simulink model "gm_uz_pmsm_model_9ph_21b_all_double_vnl"  (R2021b)
settings: Solver=FixedStepAuto  StartTime=0.0  StopTime=0.8  RelTol=1e-3
PreLoadFcn:
  | uz_pmsm_model_9ph_init_parameter
undefined symbols (not defined in the file or in its folder): a, b, c, friction_coefficient, inertia, k_i_d, k_i_q, k_p_d, k_p_q, Kpd, L_d, L_o1, L_o2, L_q, L_x1, L_x2, L_y1, L_y2, L_zero, polepair, psi_pm, R_1, static_friction_torque, Tnd, ts
libraries: hdlsllib x91, simulink x46, hdlmdlgenlib x17, dspsigops x7, slpidlib x2, spsAlphaBetaZerotodq0Lib x1, pid_lib x1, spsdq0toAlphaBetaZeroLib x1
(part 7 of 7)

== system gm_uz_pmsm_model_9ph_21b_all_double_vnl/uz_pmsm_model_9ph/abc_to_dq/abc_to_dq/_adder_MultiplyAdd74 ==
  in0 : Inport  OutDataTypeStr=fixdt(1, 18, 17)  SampleTime=1e-08
  in1 : Inport  Port=2  OutDataTypeStr=fixdt(1, 25, 12)  SampleTime=1e-08
  in2 : Inport  Port=3  OutDataTypeStr=fixdt(1, 25, 12)  SampleTime=1e-08
  globalSchedule : EnablePort  OutDataTypeStr=boolean
  HwModeRegister : Delay  DelayLength=double(1)  InitialCondition=0
  HwModeRegister1 : Delay  DelayLength=double(1)  InitialCondition=0
  HwModeRegister2 : Delay  DelayLength=double(1)  InitialCondition=0
  PipelineRegister : Delay  DelayLength=double(2)  InitialCondition=0
  _adder_MultiplyAdd : hdlsllib/HDL Operations/Multiply-Add  Function=c+(a.*b)  datatype=fixdt(1, 44, 29)  DoSatur=off  FMA=off
      settings: SourceProductBaseCode=SL
  out0 : Outport  OutDataTypeStr=fixdt(1, 44, 29)  SampleTime=1e-08  InitialOutput=0
  wires:
  HwModeRegister2/1 -> _adder_MultiplyAdd/3
  HwModeRegister1/1 -> _adder_MultiplyAdd/2
  HwModeRegister/1 -> _adder_MultiplyAdd/1
  _adder_MultiplyAdd/1 -> PipelineRegister/1
  in2/1 -> HwModeRegister2/1
  in1/1 -> HwModeRegister1/1
  in0/1 -> HwModeRegister/1
  PipelineRegister/1 -> out0/1

== system gm_uz_pmsm_model_9ph_21b_all_double_vnl/uz_pmsm_model_9ph/abc_to_dq/abc_to_dq/_adder_MultiplyAdd75 ==
  in0 : Inport  OutDataTypeStr=fixdt(1, 18, 17)  SampleTime=1e-08
  in1 : Inport  Port=2  OutDataTypeStr=fixdt(1, 25, 12)  SampleTime=1e-08
  in2 : Inport  Port=3  OutDataTypeStr=fixdt(1, 25, 12)  SampleTime=1e-08
  globalSchedule : EnablePort  OutDataTypeStr=boolean
  HwModeRegister : Delay  DelayLength=double(1)  InitialCondition=0
  HwModeRegister1 : Delay  DelayLength=double(1)  InitialCondition=0
  HwModeRegister2 : Delay  DelayLength=double(1)  InitialCondition=0
  PipelineRegister : Delay  DelayLength=double(2)  InitialCondition=0
  _adder_MultiplyAdd : hdlsllib/HDL Operations/Multiply-Add  Function=c+(a.*b)  datatype=fixdt(1, 44, 29)  DoSatur=off  FMA=off
      settings: SourceProductBaseCode=SL
  out0 : Outport  OutDataTypeStr=fixdt(1, 44, 29)  SampleTime=1e-08  InitialOutput=0
  wires:
  HwModeRegister2/1 -> _adder_MultiplyAdd/3
  HwModeRegister1/1 -> _adder_MultiplyAdd/2
  HwModeRegister/1 -> _adder_MultiplyAdd/1
  _adder_MultiplyAdd/1 -> PipelineRegister/1
  in2/1 -> HwModeRegister2/1
  in1/1 -> HwModeRegister1/1
  in0/1 -> HwModeRegister/1
  PipelineRegister/1 -> out0/1

== system gm_uz_pmsm_model_9ph_21b_all_double_vnl/uz_pmsm_model_9ph/abc_to_dq/abc_to_dq/_adder_MultiplyAdd76 ==
  in0 : Inport  OutDataTypeStr=fixdt(1, 18, 17)  SampleTime=1e-08
  in1 : Inport  Port=2  OutDataTypeStr=fixdt(1, 25, 12)  SampleTime=1e-08
  in2 : Inport  Port=3  OutDataTypeStr=fixdt(1, 25, 12)  SampleTime=1e-08
  globalSchedule : EnablePort  OutDataTypeStr=boolean
  HwModeRegister : Delay  DelayLength=double(1)  InitialCondition=0
  HwModeRegister1 : Delay  DelayLength=double(1)  InitialCondition=0
  HwModeRegister2 : Delay  DelayLength=double(1)  InitialCondition=0
  PipelineRegister : Delay  DelayLength=double(2)  InitialCondition=0
  _adder_MultiplyAdd : hdlsllib/HDL Operations/Multiply-Add  Function=c+(a.*b)  datatype=fixdt(1, 44, 29)  DoSatur=off  FMA=off
      settings: SourceProductBaseCode=SL
  out0 : Outport  OutDataTypeStr=fixdt(1, 44, 29)  SampleTime=1e-08  InitialOutput=0
  wires:
  HwModeRegister2/1 -> _adder_MultiplyAdd/3
  HwModeRegister1/1 -> _adder_MultiplyAdd/2
  HwModeRegister/1 -> _adder_MultiplyAdd/1
  _adder_MultiplyAdd/1 -> PipelineRegister/1
  in2/1 -> HwModeRegister2/1
  in1/1 -> HwModeRegister1/1
  in0/1 -> HwModeRegister/1
  PipelineRegister/1 -> out0/1

== system gm_uz_pmsm_model_9ph_21b_all_double_vnl/uz_pmsm_model_9ph/abc_to_dq/abc_to_dq/_adder_MultiplyAdd77 ==
  in0 : Inport  OutDataTypeStr=fixdt(1, 18, 17)  SampleTime=1e-08
  in1 : Inport  Port=2  OutDataTypeStr=fixdt(1, 25, 12)  SampleTime=1e-08
  in2 : Inport  Port=3  OutDataTypeStr=fixdt(1, 25, 12)  SampleTime=1e-08
  globalSchedule : EnablePort  OutDataTypeStr=boolean
  HwModeRegister : Delay  DelayLength=double(1)  InitialCondition=0
  HwModeRegister1 : Delay  DelayLength=double(1)  InitialCondition=0
  HwModeRegister2 : Delay  DelayLength=double(1)  InitialCondition=0
  PipelineRegister : Delay  DelayLength=double(2)  InitialCondition=0
  _adder_MultiplyAdd : hdlsllib/HDL Operations/Multiply-Add  Function=c+(a.*b)  datatype=fixdt(1, 44, 29)  DoSatur=off  FMA=off
      settings: SourceProductBaseCode=SL
  out0 : Outport  OutDataTypeStr=fixdt(1, 44, 29)  SampleTime=1e-08  InitialOutput=0
  wires:
  HwModeRegister2/1 -> _adder_MultiplyAdd/3
  HwModeRegister1/1 -> _adder_MultiplyAdd/2
  HwModeRegister/1 -> _adder_MultiplyAdd/1
  _adder_MultiplyAdd/1 -> PipelineRegister/1
  in2/1 -> HwModeRegister2/1
  in1/1 -> HwModeRegister1/1
  in0/1 -> HwModeRegister/1
  PipelineRegister/1 -> out0/1

== system gm_uz_pmsm_model_9ph_21b_all_double_vnl/uz_pmsm_model_9ph/abc_to_dq/abc_to_dq/_adder_MultiplyAdd78 ==
  in0 : Inport  OutDataTypeStr=fixdt(1, 18, 17)  SampleTime=1e-08
  in1 : Inport  Port=2  OutDataTypeStr=fixdt(1, 25, 12)  SampleTime=1e-08
  in2 : Inport  Port=3  OutDataTypeStr=fixdt(1, 25, 12)  SampleTime=1e-08
  globalSchedule : EnablePort  OutDataTypeStr=boolean
  HwModeRegister : Delay  DelayLength=double(1)  InitialCondition=0
  HwModeRegister1 : Delay  DelayLength=double(1)  InitialCondition=0
  HwModeRegister2 : Delay  DelayLength=double(1)  InitialCondition=0
  PipelineRegister : Delay  DelayLength=double(2)  InitialCondition=0
  _adder_MultiplyAdd : hdlsllib/HDL Operations/Multiply-Add  Function=c+(a.*b)  datatype=fixdt(1, 44, 29)  DoSatur=off  FMA=off
      settings: SourceProductBaseCode=SL
  out0 : Outport  OutDataTypeStr=fixdt(1, 44, 29)  SampleTime=1e-08  InitialOutput=0
  wires:
  HwModeRegister2/1 -> _adder_MultiplyAdd/3
  HwModeRegister1/1 -> _adder_MultiplyAdd/2
  HwModeRegister/1 -> _adder_MultiplyAdd/1
  _adder_MultiplyAdd/1 -> PipelineRegister/1
  in2/1 -> HwModeRegister2/1
  in1/1 -> HwModeRegister1/1
  in0/1 -> HwModeRegister/1
  PipelineRegister/1 -> out0/1

== system gm_uz_pmsm_model_9ph_21b_all_double_vnl/uz_pmsm_model_9ph/abc_to_dq/abc_to_dq/_adder_MultiplyAdd79 ==
  in0 : Inport  OutDataTypeStr=fixdt(1, 18, 17)  SampleTime=1e-08
  in1 : Inport  Port=2  OutDataTypeStr=fixdt(1, 25, 12)  SampleTime=1e-08
  in2 : Inport  Port=3  OutDataTypeStr=fixdt(1, 25, 12)  SampleTime=1e-08
  globalSchedule : EnablePort  OutDataTypeStr=boolean
  HwModeRegister : Delay  DelayLength=double(1)  InitialCondition=0
  HwModeRegister1 : Delay  DelayLength=double(1)  InitialCondition=0
  HwModeRegister2 : Delay  DelayLength=double(1)  InitialCondition=0
  PipelineRegister : Delay  DelayLength=double(2)  InitialCondition=0
  _adder_MultiplyAdd : hdlsllib/HDL Operations/Multiply-Add  Function=c+(a.*b)  datatype=fixdt(1, 44, 29)  DoSatur=off  FMA=off
      settings: SourceProductBaseCode=SL
  out0 : Outport  OutDataTypeStr=fixdt(1, 44, 29)  SampleTime=1e-08  InitialOutput=0
  wires:
  HwModeRegister2/1 -> _adder_MultiplyAdd/3
  HwModeRegister1/1 -> _adder_MultiplyAdd/2
  HwModeRegister/1 -> _adder_MultiplyAdd/1
  _adder_MultiplyAdd/1 -> PipelineRegister/1
  in2/1 -> HwModeRegister2/1
  in1/1 -> HwModeRegister1/1
  in0/1 -> HwModeRegister/1
  PipelineRegister/1 -> out0/1

== system gm_uz_pmsm_model_9ph_21b_all_double_vnl/uz_pmsm_model_9ph/abc_to_dq/abc_to_dq/_adder_MultiplyAdd8 ==
  in0 : Inport  OutDataTypeStr=fixdt(1, 18, 17)  SampleTime=1e-08
  in1 : Inport  Port=2  OutDataTypeStr=fixdt(1, 25, 12)  SampleTime=1e-08
  in2 : Inport  Port=3  OutDataTypeStr=fixdt(1, 25, 12)  SampleTime=1e-08
  globalSchedule : EnablePort  OutDataTypeStr=boolean
  HwModeRegister : Delay  DelayLength=double(1)  InitialCondition=0
  HwModeRegister1 : Delay  DelayLength=double(1)  InitialCondition=0
  HwModeRegister2 : Delay  DelayLength=double(1)  InitialCondition=0
  PipelineRegister : Delay  DelayLength=double(2)  InitialCondition=0
  _adder_MultiplyAdd : hdlsllib/HDL Operations/Multiply-Add  Function=c+(a.*b)  datatype=fixdt(1, 44, 29)  DoSatur=off  FMA=off
      settings: SourceProductBaseCode=SL
  out0 : Outport  OutDataTypeStr=fixdt(1, 44, 29)  SampleTime=1e-08  InitialOutput=0
  wires:
  HwModeRegister2/1 -> _adder_MultiplyAdd/3
  HwModeRegister1/1 -> _adder_MultiplyAdd/2
  HwModeRegister/1 -> _adder_MultiplyAdd/1
  _adder_MultiplyAdd/1 -> PipelineRegister/1
  in2/1 -> HwModeRegister2/1
  in1/1 -> HwModeRegister1/1
  in0/1 -> HwModeRegister/1
  PipelineRegister/1 -> out0/1

== system gm_uz_pmsm_model_9ph_21b_all_double_vnl/uz_pmsm_model_9ph/abc_to_dq/abc_to_dq/_adder_MultiplyAdd80 ==
  in0 : Inport  OutDataTypeStr=fixdt(1, 18, 17)  SampleTime=1e-08
  in1 : Inport  Port=2  OutDataTypeStr=fixdt(1, 25, 12)  SampleTime=1e-08
  in2 : Inport  Port=3  OutDataTypeStr=fixdt(1, 25, 12)  SampleTime=1e-08
  globalSchedule : EnablePort  OutDataTypeStr=boolean
  HwModeRegister : Delay  DelayLength=double(1)  InitialCondition=0
  HwModeRegister1 : Delay  DelayLength=double(1)  InitialCondition=0
  HwModeRegister2 : Delay  DelayLength=double(1)  InitialCondition=0
  PipelineRegister : Delay  DelayLength=double(2)  InitialCondition=0
  _adder_MultiplyAdd : hdlsllib/HDL Operations/Multiply-Add  Function=c+(a.*b)  datatype=fixdt(1, 44, 29)  DoSatur=off  FMA=off
      settings: SourceProductBaseCode=SL
  out0 : Outport  OutDataTypeStr=fixdt(1, 44, 29)  SampleTime=1e-08  InitialOutput=0
  wires:
  HwModeRegister2/1 -> _adder_MultiplyAdd/3
  HwModeRegister1/1 -> _adder_MultiplyAdd/2
  HwModeRegister/1 -> _adder_MultiplyAdd/1
  _adder_MultiplyAdd/1 -> PipelineRegister/1
  in2/1 -> HwModeRegister2/1
  in1/1 -> HwModeRegister1/1
  in0/1 -> HwModeRegister/1
  PipelineRegister/1 -> out0/1

== system gm_uz_pmsm_model_9ph_21b_all_double_vnl/uz_pmsm_model_9ph/abc_to_dq/abc_to_dq/_adder_MultiplyAdd9 ==
  in0 : Inport  OutDataTypeStr=fixdt(1, 18, 17)  SampleTime=1e-08
  in1 : Inport  Port=2  OutDataTypeStr=fixdt(1, 25, 12)  SampleTime=1e-08
  in2 : Inport  Port=3  OutDataTypeStr=fixdt(1, 25, 12)  SampleTime=1e-08
  globalSchedule : EnablePort  OutDataTypeStr=boolean
  HwModeRegister : Delay  DelayLength=double(1)  InitialCondition=0
  HwModeRegister1 : Delay  DelayLength=double(1)  InitialCondition=0
  HwModeRegister2 : Delay  DelayLength=double(1)  InitialCondition=0
  PipelineRegister : Delay  DelayLength=double(2)  InitialCondition=0
  _adder_MultiplyAdd : hdlsllib/HDL Operations/Multiply-Add  Function=c+(a.*b)  datatype=fixdt(1, 44, 29)  DoSatur=off  FMA=off
      settings: SourceProductBaseCode=SL
  out0 : Outport  OutDataTypeStr=fixdt(1, 44, 29)  SampleTime=1e-08  InitialOutput=0
  wires:
  HwModeRegister2/1 -> _adder_MultiplyAdd/3
  HwModeRegister1/1 -> _adder_MultiplyAdd/2
  HwModeRegister/1 -> _adder_MultiplyAdd/1
  _adder_MultiplyAdd/1 -> PipelineRegister/1
  in2/1 -> HwModeRegister2/1
  in1/1 -> HwModeRegister1/1
  in0/1 -> HwModeRegister/1
  PipelineRegister/1 -> out0/1

== system gm_uz_pmsm_model_9ph_21b_all_double_vnl/uz_pmsm_model_9ph/abc_to_dq/abc_to_dq/crp_temp_MAC ==
  in0 : Inport  OutDataTypeStr=fixdt(1, 18, 16)  PortDimensions=[9 1]  SampleTime=1e-08
  in1 : Inport  Port=2  OutDataTypeStr=fixdt(1, 25, 12)  PortDimensions=[9]  SampleTime=1e-08
  globalSchedule : EnablePort  OutDataTypeStr=boolean
  PipelineRegister : Delay  DelayLength=double(8)  InitialCondition=0
  t : hdlsllib/HDL Operations/Multiply-Accumulate  opMode=Vector  initValueSetting=Dialog  initValue=0  initValueSetting2=Dialog  initValue2=0  initValueSetting3=Dialog  initValue3=0  num_samples=2  RndMeth2=Floor  RndMeth3=Floor  OutDataTypeStr=fixdt(1, 25, 12)  datatype2=Inherit: Inherit via back propagation  datatype3=Inherit: Inherit via back propagation  validOut=on  endInandOut=on  startOut=on  countOut=on  dim=-1  DoSatur=off  parallel=off
      settings: SourceProductBaseCode=SL
  out0 : Outport  OutDataTypeStr=fixdt(1, 25, 12)  SampleTime=1e-08  InitialOutput=0
  wires:
  t/1 -> PipelineRegister/1
  in1/1 -> t/2
  in0/1 -> t/1
  PipelineRegister/1 -> out0/1

== system gm_uz_pmsm_model_9ph_21b_all_double_vnl/uz_pmsm_model_9ph/abc_to_dq/abc_to_dq/crp_temp_MAC1 ==
  in0 : Inport  OutDataTypeStr=fixdt(1, 18, 16)  PortDimensions=[9 1]  SampleTime=1e-08
  in1 : Inport  Port=2  OutDataTypeStr=fixdt(1, 25, 12)  PortDimensions=[9]  SampleTime=1e-08
  globalSchedule : EnablePort  OutDataTypeStr=boolean
  PipelineRegister : Delay  DelayLength=double(8)  InitialCondition=0
  t : hdlsllib/HDL Operations/Multiply-Accumulate  opMode=Vector  initValueSetting=Dialog  initValue=0  initValueSetting2=Dialog  initValue2=0  initValueSetting3=Dialog  initValue3=0  num_samples=2  RndMeth2=Floor  RndMeth3=Floor  OutDataTypeStr=fixdt(1, 25, 12)  datatype2=Inherit: Inherit via back propagation  datatype3=Inherit: Inherit via back propagation  validOut=on  endInandOut=on  startOut=on  countOut=on  dim=-1  DoSatur=off  parallel=off
      settings: SourceProductBaseCode=SL
  out0 : Outport  OutDataTypeStr=fixdt(1, 25, 12)  SampleTime=1e-08  InitialOutput=0
  wires:
  t/1 -> PipelineRegister/1
  in1/1 -> t/2
  in0/1 -> t/1
  PipelineRegister/1 -> out0/1

== system gm_uz_pmsm_model_9ph_21b_all_double_vnl/uz_pmsm_model_9ph/abc_to_dq/abc_to_dq/crp_temp_MAC2 ==
  in0 : Inport  OutDataTypeStr=fixdt(1, 18, 16)  PortDimensions=[9 1]  SampleTime=1e-08
  in1 : Inport  Port=2  OutDataTypeStr=fixdt(1, 25, 12)  PortDimensions=[9]  SampleTime=1e-08
  globalSchedule : EnablePort  OutDataTypeStr=boolean
  PipelineRegister : Delay  DelayLength=double(8)  InitialCondition=0
  t : hdlsllib/HDL Operations/Multiply-Accumulate  opMode=Vector  initValueSetting=Dialog  initValue=0  initValueSetting2=Dialog  initValue2=0  initValueSetting3=Dialog  initValue3=0  num_samples=2  RndMeth2=Floor  RndMeth3=Floor  OutDataTypeStr=fixdt(1, 25, 12)  datatype2=Inherit: Inherit via back propagation  datatype3=Inherit: Inherit via back propagation  validOut=on  endInandOut=on  startOut=on  countOut=on  dim=-1  DoSatur=off  parallel=off
      settings: SourceProductBaseCode=SL
  out0 : Outport  OutDataTypeStr=fixdt(1, 25, 12)  SampleTime=1e-08  InitialOutput=0
  wires:
  t/1 -> PipelineRegister/1
  in1/1 -> t/2
  in0/1 -> t/1
  PipelineRegister/1 -> out0/1

== system gm_uz_pmsm_model_9ph_21b_all_double_vnl/uz_pmsm_model_9ph/abc_to_dq/abc_to_dq/crp_temp_MAC3 ==
  in0 : Inport  OutDataTypeStr=fixdt(1, 18, 16)  PortDimensions=[9 1]  SampleTime=1e-08
  in1 : Inport  Port=2  OutDataTypeStr=fixdt(1, 25, 12)  PortDimensions=[9]  SampleTime=1e-08
  globalSchedule : EnablePort  OutDataTypeStr=boolean
  PipelineRegister : Delay  DelayLength=double(8)  InitialCondition=0
  t : hdlsllib/HDL Operations/Multiply-Accumulate  opMode=Vector  initValueSetting=Dialog  initValue=0  initValueSetting2=Dialog  initValue2=0  initValueSetting3=Dialog  initValue3=0  num_samples=2  RndMeth2=Floor  RndMeth3=Floor  OutDataTypeStr=fixdt(1, 25, 12)  datatype2=Inherit: Inherit via back propagation  datatype3=Inherit: Inherit via back propagation  validOut=on  endInandOut=on  startOut=on  countOut=on  dim=-1  DoSatur=off  parallel=off
      settings: SourceProductBaseCode=SL
  out0 : Outport  OutDataTypeStr=fixdt(1, 25, 12)  SampleTime=1e-08  InitialOutput=0
  wires:
  t/1 -> PipelineRegister/1
  in1/1 -> t/2
  in0/1 -> t/1
  PipelineRegister/1 -> out0/1

== system gm_uz_pmsm_model_9ph_21b_all_double_vnl/uz_pmsm_model_9ph/abc_to_dq/abc_to_dq/crp_temp_MAC4 ==
  in0 : Inport  OutDataTypeStr=fixdt(1, 18, 16)  PortDimensions=[9 1]  SampleTime=1e-08
  in1 : Inport  Port=2  OutDataTypeStr=fixdt(1, 25, 12)  PortDimensions=[9]  SampleTime=1e-08
  globalSchedule : EnablePort  OutDataTypeStr=boolean
  PipelineRegister : Delay  DelayLength=double(8)  InitialCondition=0
  t : hdlsllib/HDL Operations/Multiply-Accumulate  opMode=Vector  initValueSetting=Dialog  initValue=0  initValueSetting2=Dialog  initValue2=0  initValueSetting3=Dialog  initValue3=0  num_samples=2  RndMeth2=Floor  RndMeth3=Floor  OutDataTypeStr=fixdt(1, 25, 12)  datatype2=Inherit: Inherit via back propagation  datatype3=Inherit: Inherit via back propagation  validOut=on  endInandOut=on  startOut=on  countOut=on  dim=-1  DoSatur=off  parallel=off
      settings: SourceProductBaseCode=SL
  out0 : Outport  OutDataTypeStr=fixdt(1, 25, 12)  SampleTime=1e-08  InitialOutput=0
  wires:
  t/1 -> PipelineRegister/1
  in1/1 -> t/2
  in0/1 -> t/1
  PipelineRegister/1 -> out0/1

== system gm_uz_pmsm_model_9ph_21b_all_double_vnl/uz_pmsm_model_9ph/abc_to_dq/abc_to_dq/crp_temp_MAC5 ==
  in0 : Inport  OutDataTypeStr=fixdt(1, 18, 16)  PortDimensions=[9 1]  SampleTime=1e-08
  in1 : Inport  Port=2  OutDataTypeStr=fixdt(1, 25, 12)  PortDimensions=[9]  SampleTime=1e-08
  globalSchedule : EnablePort  OutDataTypeStr=boolean
  PipelineRegister : Delay  DelayLength=double(8)  InitialCondition=0
  t : hdlsllib/HDL Operations/Multiply-Accumulate  opMode=Vector  initValueSetting=Dialog  initValue=0  initValueSetting2=Dialog  initValue2=0  initValueSetting3=Dialog  initValue3=0  num_samples=2  RndMeth2=Floor  RndMeth3=Floor  OutDataTypeStr=fixdt(1, 25, 12)  datatype2=Inherit: Inherit via back propagation  datatype3=Inherit: Inherit via back propagation  validOut=on  endInandOut=on  startOut=on  countOut=on  dim=-1  DoSatur=off  parallel=off
      settings: SourceProductBaseCode=SL
  out0 : Outport  OutDataTypeStr=fixdt(1, 25, 12)  SampleTime=1e-08  InitialOutput=0
  wires:
  t/1 -> PipelineRegister/1
  in1/1 -> t/2
  in0/1 -> t/1
  PipelineRegister/1 -> out0/1

== system gm_uz_pmsm_model_9ph_21b_all_double_vnl/uz_pmsm_model_9ph/abc_to_dq/abc_to_dq/crp_temp_MAC6 ==
  in0 : Inport  OutDataTypeStr=fixdt(1, 18, 16)  PortDimensions=[9 1]  SampleTime=1e-08
  in1 : Inport  Port=2  OutDataTypeStr=fixdt(1, 25, 12)  PortDimensions=[9]  SampleTime=1e-08
  globalSchedule : EnablePort  OutDataTypeStr=boolean
  PipelineRegister : Delay  DelayLength=double(8)  InitialCondition=0
  t : hdlsllib/HDL Operations/Multiply-Accumulate  opMode=Vector  initValueSetting=Dialog  initValue=0  initValueSetting2=Dialog  initValue2=0  initValueSetting3=Dialog  initValue3=0  num_samples=2  RndMeth2=Floor  RndMeth3=Floor  OutDataTypeStr=fixdt(1, 25, 12)  datatype2=Inherit: Inherit via back propagation  datatype3=Inherit: Inherit via back propagation  validOut=on  endInandOut=on  startOut=on  countOut=on  dim=-1  DoSatur=off  parallel=off
      settings: SourceProductBaseCode=SL
  out0 : Outport  OutDataTypeStr=fixdt(1, 25, 12)  SampleTime=1e-08  InitialOutput=0
  wires:
  t/1 -> PipelineRegister/1
  in1/1 -> t/2
  in0/1 -> t/1
  PipelineRegister/1 -> out0/1

== system gm_uz_pmsm_model_9ph_21b_all_double_vnl/uz_pmsm_model_9ph/abc_to_dq/abc_to_dq/crp_temp_MAC7 ==
  in0 : Inport  OutDataTypeStr=fixdt(1, 18, 16)  PortDimensions=[9 1]  SampleTime=1e-08
  in1 : Inport  Port=2  OutDataTypeStr=fixdt(1, 25, 12)  PortDimensions=[9]  SampleTime=1e-08
  globalSchedule : EnablePort  OutDataTypeStr=boolean
  PipelineRegister : Delay  DelayLength=double(8)  InitialCondition=0
  t : hdlsllib/HDL Operations/Multiply-Accumulate  opMode=Vector  initValueSetting=Dialog  initValue=0  initValueSetting2=Dialog  initValue2=0  initValueSetting3=Dialog  initValue3=0  num_samples=2  RndMeth2=Floor  RndMeth3=Floor  OutDataTypeStr=fixdt(1, 25, 12)  datatype2=Inherit: Inherit via back propagation  datatype3=Inherit: Inherit via back propagation  validOut=on  endInandOut=on  startOut=on  countOut=on  dim=-1  DoSatur=off  parallel=off
      settings: SourceProductBaseCode=SL
  out0 : Outport  OutDataTypeStr=fixdt(1, 25, 12)  SampleTime=1e-08  InitialOutput=0
  wires:
  t/1 -> PipelineRegister/1
  in1/1 -> t/2
  in0/1 -> t/1
  PipelineRegister/1 -> out0/1

== system gm_uz_pmsm_model_9ph_21b_all_double_vnl/uz_pmsm_model_9ph/abc_to_dq/abc_to_dq/crp_temp_MAC8 ==
  in0 : Inport  OutDataTypeStr=fixdt(1, 18, 16)  PortDimensions=[9 1]  SampleTime=1e-08
  in1 : Inport  Port=2  OutDataTypeStr=fixdt(1, 25, 12)  PortDimensions=[9]  SampleTime=1e-08
  globalSchedule : EnablePort  OutDataTypeStr=boolean
  PipelineRegister : Delay  DelayLength=double(8)  InitialCondition=0
  t : hdlsllib/HDL Operations/Multiply-Accumulate  opMode=Vector  initValueSetting=Dialog  initValue=0  initValueSetting2=Dialog  initValue2=0  initValueSetting3=Dialog  initValue3=0  num_samples=2  RndMeth2=Floor  RndMeth3=Floor  OutDataTypeStr=fixdt(1, 25, 12)  datatype2=Inherit: Inherit via back propagation  datatype3=Inherit: Inherit via back propagation  validOut=on  endInandOut=on  startOut=on  countOut=on  dim=-1  DoSatur=off  parallel=off
      settings: SourceProductBaseCode=SL
  out0 : Outport  OutDataTypeStr=fixdt(1, 25, 12)  SampleTime=1e-08  InitialOutput=0
  wires:
  t/1 -> PipelineRegister/1
  in1/1 -> t/2
  in0/1 -> t/1
  PipelineRegister/1 -> out0/1

== system gm_uz_pmsm_model_9ph_21b_all_double_vnl/uz_pmsm_model_9ph/abc_to_dq/abc_to_dq/t19 ==
  in0 : Inport
  ColVec1 : Selector  NumberOfDimensions=2  IndexOptions=Select all,Index vector (dialog)  Indices=1,1  OutputSizes=1,1
  ColVec2 : Selector  NumberOfDimensions=2  IndexOptions=Select all,Index vector (dialog)  Indices=1,2  OutputSizes=1,1
  ColVec3 : Selector  NumberOfDimensions=2  IndexOptions=Select all,Index vector (dialog)  Indices=1,3  OutputSizes=1,1
  ColVec4 : Selector  NumberOfDimensions=2  IndexOptions=Select all,Index vector (dialog)  Indices=1,4  OutputSizes=1,1
  ColVec5 : Selector  NumberOfDimensions=2  IndexOptions=Select all,Index vector (dialog)  Indices=1,5  OutputSizes=1,1
  ColVec6 : Selector  NumberOfDimensions=2  IndexOptions=Select all,Index vector (dialog)  Indices=1,6  OutputSizes=1,1
  ColVec7 : Selector  NumberOfDimensions=2  IndexOptions=Select all,Index vector (dialog)  Indices=1,7  OutputSizes=1,1
  ColVec8 : Selector  NumberOfDimensions=2  IndexOptions=Select all,Index vector (dialog)  Indices=1,8  OutputSizes=1,1
  ColVec9 : Selector  NumberOfDimensions=2  IndexOptions=Select all,Index vector (dialog)  Indices=1,9  OutputSizes=1,1
  out0 : Outport
  out1 : Outport  Port=2
  out2 : Outport  Port=3
  out3 : Outport  Port=4
  out4 : Outport  Port=5
  out5 : Outport  Port=6
  out6 : Outport  Port=7
  out7 : Outport  Port=8
  out8 : Outport  Port=9
  wires:
  ColVec9/1 -> out8/1
  ColVec8/1 -> out7/1
  ColVec7/1 -> out6/1
  ColVec6/1 -> out5/1
  ColVec5/1 -> out4/1
  ColVec4/1 -> out3/1
  ColVec3/1 -> out2/1
  ColVec2/1 -> out1/1
  ColVec1/1 -> out0/1
  in0/1 -> ColVec9/1, ColVec8/1, ColVec7/1, ColVec6/1, ColVec5/1, ColVec4/1, ColVec3/1, ColVec2/1, ColVec1/1

== system gm_uz_pmsm_model_9ph_21b_all_double_vnl/uz_pmsm_model_9ph/abc_to_dq/abc_to_dq/t23 ==
  in0 : Inport
  ColVec1 : Selector  NumberOfDimensions=2  IndexOptions=Select all,Index vector (dialog)  Indices=1,1  OutputSizes=1,1
  ColVec2 : Selector  NumberOfDimensions=2  IndexOptions=Select all,Index vector (dialog)  Indices=1,2  OutputSizes=1,1
  ColVec3 : Selector  NumberOfDimensions=2  IndexOptions=Select all,Index vector (dialog)  Indices=1,3  OutputSizes=1,1
  ColVec4 : Selector  NumberOfDimensions=2  IndexOptions=Select all,Index vector (dialog)  Indices=1,4  OutputSizes=1,1
  ColVec5 : Selector  NumberOfDimensions=2  IndexOptions=Select all,Index vector (dialog)  Indices=1,5  OutputSizes=1,1
  ColVec6 : Selector  NumberOfDimensions=2  IndexOptions=Select all,Index vector (dialog)  Indices=1,6  OutputSizes=1,1
  ColVec7 : Selector  NumberOfDimensions=2  IndexOptions=Select all,Index vector (dialog)  Indices=1,7  OutputSizes=1,1
  ColVec8 : Selector  NumberOfDimensions=2  IndexOptions=Select all,Index vector (dialog)  Indices=1,8  OutputSizes=1,1
  ColVec9 : Selector  NumberOfDimensions=2  IndexOptions=Select all,Index vector (dialog)  Indices=1,9  OutputSizes=1,1
  out0 : Outport
  out1 : Outport  Port=2
  out2 : Outport  Port=3
  out3 : Outport  Port=4
  out4 : Outport  Port=5
  out5 : Outport  Port=6
  out6 : Outport  Port=7
  out7 : Outport  Port=8
  out8 : Outport  Port=9
  wires:
  ColVec9/1 -> out8/1
  ColVec8/1 -> out7/1
  ColVec7/1 -> out6/1
  ColVec6/1 -> out5/1
  ColVec5/1 -> out4/1
  ColVec4/1 -> out3/1
  ColVec3/1 -> out2/1
  ColVec2/1 -> out1/1
  ColVec1/1 -> out0/1
  in0/1 -> ColVec9/1, ColVec8/1, ColVec7/1, ColVec6/1, ColVec5/1, ColVec4/1, ColVec3/1, ColVec2/1, ColVec1/1

== system gm_uz_pmsm_model_9ph_21b_all_double_vnl/uz_pmsm_model_9ph/abc_to_dq_vnl/Line-Line to Phase voltage/abc   to   alpha_beta_0 ==
  "a, b, c" : Inport  PortDimensions=3
  Gain2 : Gain  Gain=2/3  ParamDataTypeStr=fixdt(1,18,16)  SaturateOnIntegerOverflow=on  OutDataTypeStr=Inherit: Same as input
  Gain4 : Gain  Gain="[ 1   -0.5   -0.5; 0   0.5*sqrt(3)   -0.5*sqrt(3); 0.5  0.5  0.5 ]"  Multiplication=Matrix(K*u) (u vector)  ParamDataTypeStr=fixdt(1,18,16)  OutDataTypeStr=fixdt(1,25,12)  SaturateOnIntegerOverflow=on
  "alpha, beta, 0 " : Outport
  wires:
  Gain4/1 -> Gain2/1
  "a, b, c"/1 -> Gain4/1
  Gain2/1 -> "alpha, beta, 0 "/1

== system gm_uz_pmsm_model_9ph_21b_all_double_vnl/uz_pmsm_model_9ph/abc_to_dq_vnl/Line-Line to Phase voltage/alpha_beta_0   to   abc ==
  "alpha, beta, 0  " : Inport  PortDimensions=3
  Gain4 : Gain  Gain="[ 1 0 1; -0.5   0.5*sqrt(3)  1; -0.5 -0.5*sqrt(3) 1 ]"  Multiplication=Matrix(K*u) (u vector)  ParamDataTypeStr=fixdt(1,18,16)  SaturateOnIntegerOverflow=on  OutDataTypeStr=Inherit: Same as input
  "a, b, c" : Outport
  wires:
  "alpha, beta, 0  "/1 -> Gain4/1
  Gain4/1 -> "a, b, c"/1

== system gm_uz_pmsm_model_9ph_21b_all_double_vnl/uz_pmsm_model_9ph/abc_to_dq_vnl/Line-Line to Phase voltage1/abc   to   alpha_beta_0 ==
  "a, b, c" : Inport  PortDimensions=3
  Gain2 : Gain  Gain=2/3  ParamDataTypeStr=fixdt(1,18,16)  SaturateOnIntegerOverflow=on  OutDataTypeStr=Inherit: Same as input
  Gain4 : Gain  Gain="[ 1   -0.5   -0.5; 0   0.5*sqrt(3)   -0.5*sqrt(3); 0.5  0.5  0.5 ]"  Multiplication=Matrix(K*u) (u vector)  ParamDataTypeStr=fixdt(1,18,16)  OutDataTypeStr=fixdt(1,25,12)  SaturateOnIntegerOverflow=on
  "alpha, beta, 0 " : Outport
  wires:
  Gain2/1 -> "alpha, beta, 0 "/1
  "a, b, c"/1 -> Gain4/1
  Gain4/1 -> Gain2/1

== system gm_uz_pmsm_model_9ph_21b_all_double_vnl/uz_pmsm_model_9ph/abc_to_dq_vnl/Line-Line to Phase voltage1/alpha_beta_0   to   abc ==
  "alpha, beta, 0  " : Inport  PortDimensions=3
  Gain4 : Gain  Gain="[ 1 0 1; -0.5   0.5*sqrt(3)  1; -0.5 -0.5*sqrt(3) 1 ]"  Multiplication=Matrix(K*u) (u vector)  ParamDataTypeStr=fixdt(1,18,16)  SaturateOnIntegerOverflow=on  OutDataTypeStr=Inherit: Same as input
  "a, b, c" : Outport
  wires:
  Gain4/1 -> "a, b, c"/1
  "alpha, beta, 0  "/1 -> Gain4/1

== system gm_uz_pmsm_model_9ph_21b_all_double_vnl/uz_pmsm_model_9ph/abc_to_dq_vnl/Line-Line to Phase voltage2/abc   to   alpha_beta_0 ==
  "a, b, c" : Inport  PortDimensions=3
  Gain2 : Gain  Gain=2/3  ParamDataTypeStr=fixdt(1,18,16)  SaturateOnIntegerOverflow=on  OutDataTypeStr=Inherit: Same as input
  Gain4 : Gain  Gain="[ 1   -0.5   -0.5; 0   0.5*sqrt(3)   -0.5*sqrt(3); 0.5  0.5  0.5 ]"  Multiplication=Matrix(K*u) (u vector)  ParamDataTypeStr=fixdt(1,18,16)  OutDataTypeStr=fixdt(1,25,12)  SaturateOnIntegerOverflow=on
  "alpha, beta, 0 " : Outport
  wires:
  Gain4/1 -> Gain2/1
  "a, b, c"/1 -> Gain4/1
  Gain2/1 -> "alpha, beta, 0 "/1

== system gm_uz_pmsm_model_9ph_21b_all_double_vnl/uz_pmsm_model_9ph/abc_to_dq_vnl/Line-Line to Phase voltage2/alpha_beta_0   to   abc ==
  "alpha, beta, 0  " : Inport  PortDimensions=3
  Gain4 : Gain  Gain="[ 1 0 1; -0.5   0.5*sqrt(3)  1; -0.5 -0.5*sqrt(3) 1 ]"  Multiplication=Matrix(K*u) (u vector)  ParamDataTypeStr=fixdt(1,18,16)  SaturateOnIntegerOverflow=on  OutDataTypeStr=Inherit: Same as input
  "a, b, c" : Outport
  wires:
  "alpha, beta, 0  "/1 -> Gain4/1
  Gain4/1 -> "a, b, c"/1

== system gm_uz_pmsm_model_9ph_21b_all_double_vnl/uz_pmsm_model_9ph/dq_model_9ph/mechanical_system/integrator ==
  in : Inport
  reset : Inport  Port=2
  Delay1 : Delay  DelayLength=1  ExternalReset=Level
      settings: InputPortMap=u0,r5
  Gain : Gain  Gain=ts  OutDataTypeStr=Inherit: Same as input
  Sum3 : Sum  Inputs=|++  OutDataTypeStr=Inherit: Same as first input
  outt : Outport
  wires:
  Sum3/1 -> Delay1/1
  Delay1/1 -> Sum3/2, outt/1
  in/1 -> Gain/1
  Gain/1 -> Sum3/1
  reset/1 -> Delay1/2

== system gm_uz_pmsm_model_9ph_21b_all_double_vnl/uz_pmsm_model_9ph/dq_model_9ph/pmsm/integrator ==
  in : Inport
  reset : Inport  Port=2
  Delay1 : Delay  DelayLength=1  ExternalReset=Level
      settings: InputPortMap=u0,r5
  Gain : Gain  Gain=ts  OutDataTypeStr=Inherit: Same as input
  Sum3 : Sum  Inputs=|++  OutDataTypeStr=Inherit: Same as first input
  outt : Outport
  wires:
  Sum3/1 -> Delay1/1
  Delay1/1 -> Sum3/2, outt/1
  in/1 -> Gain/1
  Gain/1 -> Sum3/1
  reset/1 -> Delay1/2

== system gm_uz_pmsm_model_9ph_21b_all_double_vnl/uz_pmsm_model_9ph/dq_model_9ph/pmsm/integrator1 ==
  in : Inport
  reset : Inport  Port=2
  Delay1 : Delay  DelayLength=1  ExternalReset=Level
      settings: InputPortMap=u0,r5
  Gain : Gain  Gain=ts  OutDataTypeStr=Inherit: Same as input
  Sum3 : Sum  Inputs=|++  OutDataTypeStr=Inherit: Same as first input
  outt : Outport
  wires:
  Sum3/1 -> Delay1/1
  Delay1/1 -> Sum3/2, outt/1
  in/1 -> Gain/1
  Gain/1 -> Sum3/1
  reset/1 -> Delay1/2

== system gm_uz_pmsm_model_9ph_21b_all_double_vnl/uz_pmsm_model_9ph/dq_model_9ph/pmsm/integrator2 ==
  in : Inport
  reset : Inport  Port=2
  Delay1 : Delay  DelayLength=1  ExternalReset=Level
      settings: InputPortMap=u0,r5
  Gain : Gain  Gain=ts  OutDataTypeStr=Inherit: Same as input
  Sum3 : Sum  Inputs=|++  OutDataTypeStr=Inherit: Same as first input
  outt : Outport
  wires:
  Sum3/1 -> Delay1/1
  Delay1/1 -> Sum3/2, outt/1
  in/1 -> Gain/1
  Gain/1 -> Sum3/1
  reset/1 -> Delay1/2

== system gm_uz_pmsm_model_9ph_21b_all_double_vnl/uz_pmsm_model_9ph/dq_model_9ph/pmsm/integrator3 ==
  in : Inport
  reset : Inport  Port=2
  Delay1 : Delay  DelayLength=1  ExternalReset=Level
      settings: InputPortMap=u0,r5
  Gain : Gain  Gain=ts  OutDataTypeStr=Inherit: Same as input
  Sum3 : Sum  Inputs=|++  OutDataTypeStr=Inherit: Same as first input
  outt : Outport
  wires:
  Sum3/1 -> Delay1/1
  Delay1/1 -> Sum3/2, outt/1
  in/1 -> Gain/1
  Gain/1 -> Sum3/1
  reset/1 -> Delay1/2

== system gm_uz_pmsm_model_9ph_21b_all_double_vnl/uz_pmsm_model_9ph/dq_model_9ph/pmsm/integrator4 ==
  in : Inport
  reset : Inport  Port=2
  Delay1 : Delay  DelayLength=1  ExternalReset=Level
      settings: InputPortMap=u0,r5
  Gain : Gain  Gain=ts  OutDataTypeStr=Inherit: Same as input
  Sum3 : Sum  Inputs=|++  OutDataTypeStr=Inherit: Same as first input
  outt : Outport
  wires:
  Sum3/1 -> Delay1/1
  Delay1/1 -> Sum3/2, outt/1
  in/1 -> Gain/1
  Gain/1 -> Sum3/1
  reset/1 -> Delay1/2

== system gm_uz_pmsm_model_9ph_21b_all_double_vnl/uz_pmsm_model_9ph/dq_model_9ph/pmsm/integrator5 ==
  in : Inport
  reset : Inport  Port=2
  Delay1 : Delay  DelayLength=1  ExternalReset=Level
      settings: InputPortMap=u0,r5
  Gain : Gain  Gain=ts  OutDataTypeStr=Inherit: Same as input
  Sum3 : Sum  Inputs=|++  OutDataTypeStr=Inherit: Same as first input
  outt : Outport
  wires:
  Sum3/1 -> Delay1/1
  Delay1/1 -> Sum3/2, outt/1
  in/1 -> Gain/1
  Gain/1 -> Sum3/1
  reset/1 -> Delay1/2

== system gm_uz_pmsm_model_9ph_21b_all_double_vnl/uz_pmsm_model_9ph/dq_model_9ph/pmsm/integrator6 ==
  in : Inport
  reset : Inport  Port=2
  Delay1 : Delay  DelayLength=1  ExternalReset=Level
      settings: InputPortMap=u0,r5
  Gain : Gain  Gain=ts  OutDataTypeStr=Inherit: Same as input
  Sum3 : Sum  Inputs=|++  OutDataTypeStr=Inherit: Same as first input
  outt : Outport
  wires:
  Sum3/1 -> Delay1/1
  Delay1/1 -> Sum3/2, outt/1
  in/1 -> Gain/1
  Gain/1 -> Sum3/1
  reset/1 -> Delay1/2

== system gm_uz_pmsm_model_9ph_21b_all_double_vnl/uz_pmsm_model_9ph/dq_model_9ph/pmsm/integrator7 ==
  in : Inport
  reset : Inport  Port=2
  Delay1 : Delay  DelayLength=1  ExternalReset=Level
      settings: InputPortMap=u0,r5
  Gain : Gain  Gain=ts  OutDataTypeStr=Inherit: Same as input
  Sum3 : Sum  Inputs=|++  OutDataTypeStr=Inherit: Same as first input
  outt : Outport
  wires:
  Sum3/1 -> Delay1/1
  Delay1/1 -> Sum3/2, outt/1
  in/1 -> Gain/1
  Gain/1 -> Sum3/1
  reset/1 -> Delay1/2

== system gm_uz_pmsm_model_9ph_21b_all_double_vnl/uz_pmsm_model_9ph/dq_model_9ph/pmsm/integrator8 ==
  in : Inport
  reset : Inport  Port=2
  Delay1 : Delay  DelayLength=1  ExternalReset=Level
      settings: InputPortMap=u0,r5
  Gain : Gain  Gain=ts  OutDataTypeStr=Inherit: Same as input
  Sum3 : Sum  Inputs=|++  OutDataTypeStr=Inherit: Same as first input
  outt : Outport
  wires:
  Sum3/1 -> Delay1/1
  Delay1/1 -> Sum3/2, outt/1
  in/1 -> Gain/1
  Gain/1 -> Sum3/1
  reset/1 -> Delay1/2
